simulink model "tp2ej2c"  (R2024a)
settings: Solver=FixedStepAuto  StartTime=0.0  StopTime=10.0  FixedStep=1e-5  RelTol=1e-3
libraries: cstblocks x2
settings Model: Creator=fab  LastModifiedBy=fab

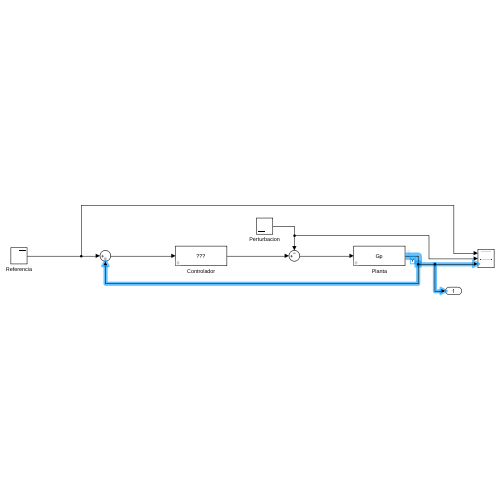
[thumbnail: Simulink's stored preview of the top-level diagram]
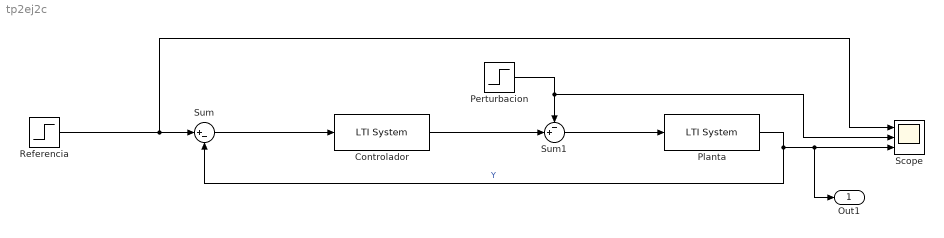
== system tp2ej2c ==
  Controlador : cstblocks/LTI System  sys=Gc  IC=[]  PadeOrder=0
  Perturbacion : Step  Time=6  After=0.2  SampleTime=0
  Planta : cstblocks/LTI System  sys=Gp  IC=[]  PadeOrder=0
  Referencia : Step  Time=0  SampleTime=0
  Scope : Scope  NumInputPorts=3
  Sum : Sum  Inputs=|+-
  Sum1 : Sum  Inputs=-+|
  Out1 : Outport
  wires:
  Referencia/1 -> Scope/1, Sum/1
  Planta/1 -> Out1/1, Scope/3, Sum/2  "Y"
  Perturbacion/1 -> Scope/2, Sum1/1
  Sum/1 -> Controlador/1
  Controlador/1 -> Sum1/2
  Sum1/1 -> Planta/1
